simulink model "fixedWingPath"  (R2023b)
settings: Solver=FixedStepAuto  StartTime=0.0  StopTime=70  FixedStep=0.01  RelTol=1e-3
model workspace: external: MATLAB File variable.m (data not in the file)
undefined symbols (not defined in the file or in its folder): DiscIntNeverNeededParam, LOGPOSX, POSY, Tgps, Tneuro, VarImu, VarNeuro
libraries: simulink x2, embmathops x2, uavalgslib x2, robotcorelib x1, uavutilslib x1
(part 2 of 2)

== matlab function fixedWingPath/Esitmateur Traj/Test/MATLAB Function2 ==
  data: a input; y0 output; b input; c input; d input; e input; f input; g input; h input; ii input; jj input; k input; l input; m input; n input; o input
function y0   = fcn(a, b, c, d, e, f, g ,h, ii, jj, k, l, m, n, o)
%temps =[0 1 2 3 4 5];
%elevation =[f e d c b a];
temps =[0 1 2 3 4 5 6 7 8 9 10 11 12 13 14];
elevation =[o n m l k jj ii h g f e d c b a];

windowSize = 15; %filtrage sur 3s
%elevation_sg = sgolayfilt(elevation, 2 ,windowSize);
elevation_smoothed = movmean(elevation, windowSize);

%weights = linspace(1, 0, windowSize);


y0 = elevation_smoothed(15);

== matlab function fixedWingPath/Esitmateur Traj1/MATLAB Function2 ==
  data: Const input; Const2 input; a input; y0 output; b input; c input; d input; e input; f input; y1 output; y2 output; y3 output; y4 output
function [y0, y1, y2, y3, y4]  = fcn(Const, Const2 ,a, b, c, d, e, f)
Tneuro = Const2;
Tgps = Const;

temps =[0 1 2 3 4 5];
elevation =[f e d c b a];
Coeff = 3;
windowSize = 3;

tempsInterp = 0:Tgps:10;
Delay = -7;

numPoints = round(Coeff);

numPoints = max(numPoints, 3);

indices = round(linspace(1 + (6-numPoints), 6, numPoints));

% Sélectionnez les points correspondants
temps = temps(indices);
elevation = elevation(indices);


elevation_smoothed = movmean(elevation, windowSize);
%elevation_smoothed = sgolayfilt(elevation, 1 ,3);
coefficients = polyfit(temps, elevation_smoothed, 1);

% Régression polynomiale d'ordre 2
interpolation = polyval(coefficients, tempsInterp);

%interpolation = spline(temps, elevation_smoothed, tempsInterp);
y0 = interpolation(7/Tgps +1-Delay);
y1 = interpolation(7/Tgps +2-Delay);
y2 = interpolation(7/Tgps +3-Delay);
y3 = interpolation(7/Tgps +4-Delay);
y4 = interpolation(7/Tgps +5-Delay);


%interpolation = interp1(temps, elevation, tempsInterp, 'spline');
%y = interpolation(20);

== matlab function fixedWingPath/Esitmateur Traj1/MATLAB Function1 ==
  data: Const input; Const2 input; a input; y0 output; b input; c input; d input; e input; f input; y1 output; y2 output; y3 output; y4 output
function [y0, y1, y2, y3, y4]  = fcn(Const, Const2 ,a, b, c, d, e, f)
Tneuro = Const2;
Tgps = Const;

temps =[0 1 2 3 4 5];
elevation =[f e d c b a];
Coeff = 3;
windowSize = 3;

tempsInterp = 0:Tgps:10;
Delay = -7;

numPoints = round(Coeff);

numPoints = max(numPoints, 3);

indices = round(linspace(1 + (6-numPoints), 6, numPoints));

% Sélectionnez les points correspondants
temps = temps(indices);
elevation = elevation(indices);


elevation_smoothed = movmean(elevation, windowSize);
%elevation_smoothed = sgolayfilt(elevation, 1 ,3);
coefficients = polyfit(temps, elevation_smoothed, 1);

% Régression polynomiale d'ordre 2
interpolation = polyval(coefficients, tempsInterp);

%interpolation = spline(temps, elevation_smoothed, tempsInterp);
y0 = interpolation(7/Tgps +1-Delay);
y1 = interpolation(7/Tgps +2-Delay);
y2 = interpolation(7/Tgps +3-Delay);
y3 = interpolation(7/Tgps +4-Delay);
y4 = interpolation(7/Tgps +5-Delay);


%interpolation = interp1(temps, elevation, tempsInterp, 'spline');
%y = interpolation(20);

== matlab function fixedWingPath/Esitmateur Traj1/Test2/MATLAB Function2 ==
  data: a input; y0 output; b input; c input; d input; e input; f input; g input; h input; ii input; jj input; k input; l input; m input; n input; o input
function y0   = fcn(a, b, c, d, e, f, g ,h, ii, jj, k, l, m, n, o)
%temps =[0 1 2 3 4 5];
%elevation =[f e d c b a];
temps =[0 1 2 3 4 5 6 7 8 9 10 11 12 13 14];
elevation =[o n m l k jj ii h g f e d c b a];

windowSize = 15; %filtrage sur 3s
%elevation_sg = sgolayfilt(elevation, 2 ,windowSize);
elevation_smoothed = movmean(elevation, windowSize);

%weights = linspace(1, 0, windowSize);


y0 = elevation_smoothed(15);

== matlab function fixedWingPath/Esitmateur Traj1/Test/MATLAB Function2 ==
  data: a input; y0 output; b input; c input; d input; e input; f input; g input; h input; ii input; jj input; k input; l input; m input; n input; o input
function y0   = fcn(a, b, c, d, e, f, g ,h, ii, jj, k, l, m, n, o)
%temps =[0 1 2 3 4 5];
%elevation =[f e d c b a];
temps =[0 1 2 3 4 5 6 7 8 9 10 11 12 13 14];
elevation =[o n m l k jj ii h g f e d c b a];

windowSize = 15; %filtrage sur 3s
%elevation_sg = sgolayfilt(elevation, 2 ,windowSize);
elevation_smoothed = movmean(elevation, windowSize);

%weights = linspace(1, 0, windowSize);


y0 = elevation_smoothed(15);

== matlab function fixedWingPath/Unidim Kalman/MATLAB Function ==
  data: MEA input; Estimation output; Et1n input; Et1 output; Emea input; Est1n input; trig input
function [Estimation, Et1] = fcn(MEA, Et1n, Emea, Est1n, trig)

Kg=Et1n/(Et1n+Emea);

if trig == 1
    Et1n = 4;
    Kg=Et1n/(Et1n+Emea);
    Est1n = 1;
end

Estimation = Est1n + Kg*[MEA - Est1n];

Et1= [1-Kg]*(Et1n);

== matlab function fixedWingPath/Esitmateur Traj/MATLAB Function2 ==
  data: Const input; Const2 input; a input; y0 output; b input; c input; d input; e input; f input; y1 output; y2 output; y3 output; y4 output
function [y0, y1, y2, y3, y4]  = fcn(Const, Const2 ,a, b, c, d, e, f)
Tneuro = Const2;
Tgps = Const;

temps =[0 1 2 3 4 5];
elevation =[f e d c b a];
Coeff = 4;
windowSize = 3;

tempsInterp = 0:Tgps:9;
Delay = -2;

numPoints = round(Coeff);

numPoints = max(numPoints, 3);

indices = round(linspace(1 + (6-numPoints), 6, numPoints));

% Sélectionnez les points correspondants
temps = temps(indices);
elevation = elevation(indices);


elevation_smoothed = movmean(elevation, windowSize);
%elevation_smoothed = sgolayfilt(elevation, 1 ,3);
coefficients = polyfit(temps, elevation_smoothed, 2);

% Régression polynomiale d'ordre 2
interpolation = polyval(coefficients, tempsInterp);

%interpolation = spline(temps, elevation_smoothed, tempsInterp);
y0 = interpolation(7/Tgps +1-Delay);
y1 = interpolation(7/Tgps +2-Delay);
y2 = interpolation(7/Tgps +3-Delay);
y3 = interpolation(7/Tgps +4-Delay);
y4 = interpolation(7/Tgps +5-Delay);


%interpolation = interp1(temps, elevation, tempsInterp, 'spline');
%y = interpolation(20);

== matlab function fixedWingPath/Subsystem/MATLAB Function ==
  data: lat1 input; distanceNord output; lon1 input; lat2 input; lon2 input; distanceEst output
function [distanceNord, distanceEst] = calculerDistanceGPS_NordEst(lat1, lon1, lat2, lon2)
    % Conversion des coordonnées en radians
    lat1 = deg2rad(lat1);
    lon1 = deg2rad(lon1);
    lat2 = deg2rad(lat2);
    lon2 = deg2rad(lon2);

    % Rayon de la Terre en mètres
    rayonTerre = 6371000;

    % Calcul des différences de coordonnées
    dlat = lat2 - lat1;
    dlon = lon2 - lon1;

    % Calcul de la distance Nord et Est
    distanceNord = rayonTerre * dlat;
    distanceEst = rayonTerre * dlon * cos((lat1 + lat2) / 2);

end

== matlab function fixedWingPath/Heading Control ==
  data: FlightState input Bus: FixedWingStateBus; UHeading input; RollAngle output size=[1 1]; e input Bus: FixedWingEnvironmentBus; PHeadingAngle parameter
function RollAngle = fcn(FlightState, UHeading, e, PHeadingAngle)
    
    Va = FlightState.AirSpeed;
    HeadingAngle = FlightState.HeadingAngle;
    FlightPathAngle = FlightState.FlightPathAngle;
    
    YawAngle = HeadingAngle - asin((1/Va)*[e.WindNorth, e.WindEast]*[-sin(HeadingAngle); cos(HeadingAngle)]);
    b = [cos(HeadingAngle)*cos(FlightPathAngle), sin(HeadingAngle)*cos(FlightPathAngle), -sin(FlightPathAngle)]*[e.WindNorth; e.WindEast; e.WindDown];
    c = [e.WindNorth, e.WindEast, e.WindDown]*[e.WindNorth; e.WindEast; e.WindDown]- Va^2;
    Vg = -b+sqrt(b^2-c);
    
    RollAngle = atan2(PHeadingAngle*angdiff(HeadingAngle,UHeading)*Vg,e.Gravity*cos(HeadingAngle-YawAngle));

== matlab function fixedWingPath/Esitmateur Traj/MATLAB Function1 ==
  data: Const input; Const2 input; a input; y0 output; b input; c input; d input; e input; f input; y1 output; y2 output; y3 output; y4 output
function [y0, y1, y2, y3, y4]  = fcn(Const, Const2 ,a, b, c, d, e, f)
Tneuro = Const2;
Tgps = Const;

temps =[0 1 2 3 4 5];
elevation =[f e d c b a];
Coeff = 4;
windowSize = 3;

tempsInterp = 0:Tgps:9;
Delay = -2;

numPoints = round(Coeff);

numPoints = max(numPoints, 3);

indices = round(linspace(1 + (6-numPoints), 6, numPoints));

% Sélectionnez les points correspondants
temps = temps(indices);
elevation = elevation(indices);


elevation_smoothed = movmean(elevation, windowSize);
%elevation_smoothed = sgolayfilt(elevation, 1 ,3);
coefficients = polyfit(temps, elevation_smoothed, 2);

% Régression polynomiale d'ordre 2
interpolation = polyval(coefficients, tempsInterp);

%interpolation = spline(temps, elevation_smoothed, tempsInterp);
y0 = interpolation(7/Tgps +1-Delay);
y1 = interpolation(7/Tgps +2-Delay);
y2 = interpolation(7/Tgps +3-Delay);
y3 = interpolation(7/Tgps +4-Delay);
y4 = interpolation(7/Tgps +5-Delay);


%interpolation = interp1(temps, elevation, tempsInterp, 'spline');
%y = interpolation(20);

== matlab function fixedWingPath/Error Visu/Esitmateur 1/MATLAB Function2 ==
  data: a input; y0 output; b input; c input; d input; e input; f input; g input; h input; ai input; aj input
function y0   = fcn(a, b, c, d, e, f, g ,h , ai, aj)
%temps =[0 1 2 3 4 5];
%elevation =[f e d c b a];
temps =[0 1 2 3 4 5 6 7 8];
elevation =[aj ai h g f e d c b a];

Delay = 0;

windowSize = 9;
elevation_smoothed = movmean(elevation, windowSize);


y0 = elevation_smoothed(7);

== matlab function fixedWingPath/2ème étage/Esitmateur 1/MATLAB Function1 ==
  data: a input; y0 output; b input; c input; d input; e input; f input; g input; h input; ai input; aj input
function y0   = fcn(a, b, c, d, e, f, g ,h , ai, aj)
%temps =[0 1 2 3 4 5];
%elevation =[f e d c b a];
temps =[0 1 2 3 4 5 6 7 8 9];
elevation =[aj ai h g f e d c b a];

Delay = 0;

windowSize = 9;
elevation_smoothed = movmean(elevation, windowSize);


y0 = elevation_smoothed(9);
